simulink model "LinearModelNoFeedback"  (R2021b)
settings: Solver=VariableStepAuto  StartTime=tStart  StopTime=tFinal  RelTol=1e-3
values from neighbouring files (symbols this model uses):
  A = [0       1 ... (first row only)    [ltdSimulationParameters.m]
  B = [0 ... (first row only)    [ltdSimulationParameters.m]
  C = [0 1]    [ltdSimulationParameters.m]
  maxTractiveEffort = 100 * 10 ^3    (= 100000)    [ltdSimulationParameters.m]
  x_0 = [x_1 x_2]'    [ltdSimulationParameters.m]
settings Model: Creator=User  LastModifiedBy=User
settings SolverCC: AlgebraicLoopSolver=TrustRegion
settings DebuggingCC: SFMachineParentedDataDiag=warning

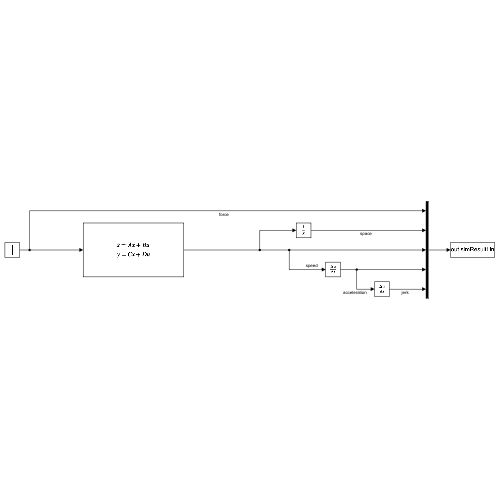
[thumbnail: Simulink's stored preview of the top-level diagram]
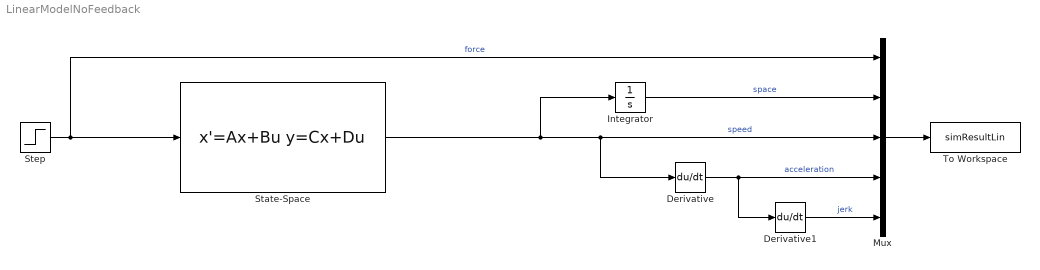
== system LinearModelNoFeedback ==
  Derivative : Derivative
  Derivative1 : Derivative
  Integrator : Integrator
  Mux : Mux  Inputs=5
  State-Space : StateSpace  A=A  B=B  C=C  D=0  InitialCondition=x_0
  Step : Step  After=maxTractiveEffort  SampleTime=0
  To Workspace : ToWorkspace  VariableName=simResultLin  SaveFormat=Structure With Time  SampleTime=-1
  wires:
  Integrator/1 -> Mux/2  "space"
  State-Space/1 -> Integrator/1, Derivative/1, Mux/3  "speed"
  Step/1 -> State-Space/1, Mux/1  "force"
  Derivative/1 -> Derivative1/1, Mux/4  "acceleration"
  Derivative1/1 -> Mux/5  "jerk"
  Mux/1 -> To Workspace/1
